simulink model "vipcodec"  (Simulink 7.7)
settings: Solver=FixedStepDiscrete  StartTime=0.0  StopTime=inf  RelTol=1e-3
undefined symbols (not defined in the file or in its folder): get, gray, M, N, rsgenpoly, sz
libraries: vipmisc x12, commutil2 x6, dspsigops x4, dspmtrx3 x4, vipsnks x3, commcnvintrlv2 x2, commblkcod2 x2, commcnvcod2 x2, viptransforms x2, viputilities x2, dspxfrm3 x2, commdigbbndam3 x2
settings Model: Creator=navan  LastModifiedBy=katsikas  CovMetricSettings=d  ExtModeAutoUpdateStatusClock=off
settings DataIOCC: SaveOutput=off  SaveTime=off  SignalLoggingName=logsOut
settings OptimizationCC: InlineParams=on  InlineInvariantSignals=on  InitFltsAndDblsToZero=on  EfficientMapNaN2IntZero=off  BufferReusableBoundary=off
settings DebuggingCC: SaveWithParameterizedLinksMsg=none  CheckExecutionContextPreStartOutputMsg=on  CheckExecutionContextRuntimeOutputMsg=on  SignalResolutionControl=TryResolveAllWithWarning  SolverPrmCheckMsg=none  MultiTaskDSMMsg=warning  MultiTaskCondExecSysMsg=none  BusObjectLabelMismatch=none  StrictBusMsg=None
settings HardwareCC: TargetBitPerLong=64  TargetBitPerPointer=64  TargetEndianess=LittleEndian  TargetWordSize=64  TargetHWDeviceType=Generic->MATLAB Host Computer  ProdEqTarget=off
settings ModelReferenceCC: UpdateModelReferenceTargets=IfOutOfDate
settings SFSimCC: SimParseCustomCode=off
settings RTWCC: IncludeERTFirstTime=on
settings GRTTargetCC: TargetFcnLib=ansi_tfl_tmw.mat

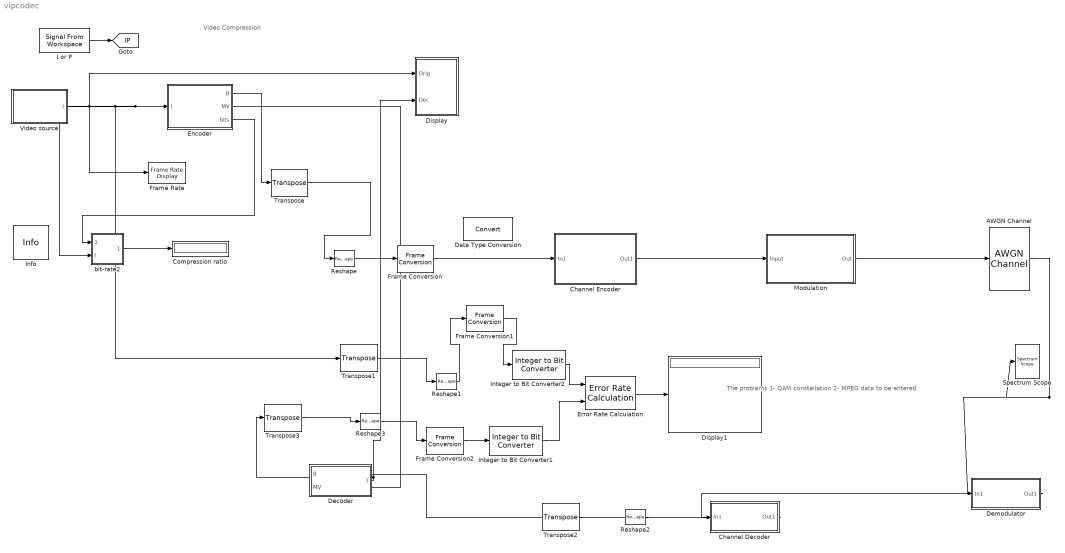
== system vipcodec ==
  note: Video Compression
  note: The problems
      | 1- QAM constellation
      | 2- MPEG data to be entered
  AWGN Channel : commchan3/AWGN Channel  SystemSampleTime=-1  InputProcessing=Inherited (this choice will be removed - see release notes)  seed=67  noiseMode="Signal to noise ratio  (SNR)"  EbNodB=10  EsNodB=10  SNRdB=10  bitsPerSym=1  Ps=1/2048  Tsym=1  variance=1
  Channel Decoder : Subsystem
  Channel Encoder : Subsystem
  Compression ratio : Display
  Data Type Conversion : DataTypeConversion
  Decoder : Subsystem
  Demodulator : Subsystem
  Display : Subsystem
  Display1 : Display
  Encoder : Subsystem
  Error Rate Calculation : commsink2/Error Rate Calculation  N=0  st_delay=0  cp_mode=Entire frame  subframe=[]  PMode=Port  WsName=ErrorVec  RsMode2=off  stop=off  numErr=100  maxBits=1e6
  Frame Conversion : FrameConversion
  Frame Conversion1 : FrameConversion
  Frame Conversion2 : FrameConversion
  Frame Rate : vipsnks/Frame Rate Display  UpdateRate=10
  I or P : dspsrcs4/Signal From Workspace  SystemSampleTime=-1  X=logical([0 0 1])  Ts=1/30  nsamps=1  OutputAfterFinalValue=Cyclic repetition  ignoreOrWarnInputAndFrameLengths=off
  Info : vipmisc/Info  SystemSampleTime=-1
  Integer to Bit Converter1 : commutil2/Integer to Bit Converter  nbits=8  signedInputValues=Unsigned  bitOrder=MSB first  outDtype=double
  Integer to Bit Converter2 : commutil2/Integer to Bit Converter  nbits=8  signedInputValues=Unsigned  bitOrder=MSB first  outDtype=double
  Modulation : Subsystem
  Reshape : Reshape  OutputDimensionality=Column vector (2-D)
  Reshape1 : Reshape  OutputDimensionality=Column vector (2-D)
  Reshape2 : Reshape  OutputDimensionality=Customize  OutputDimensions=[10,105]
  Reshape3 : Reshape  OutputDimensionality=Column vector (2-D)
  Spectrum Scope : dspsnks4/Spectrum Scope  SystemSampleTime=-1  ScopeProperties=on  Domain=Frequency  HorizSpan=1  UseBuffer=off  BufferSize=128  Overlap=64  TreatMby1Signals=One channel  inpFftLenInherit=off  FFTlength=128  numAvg=2  DisplayProperties=off  AxisGrid=on  Memory=off  FrameNumber=on  AxisLegend=off  AxisZoom=off  OpenScopeAtSimStart=on  OpenScopeImmediately=off  FigPos=get(0,'defaultfigureposition')  AxisProperties=off  XUnits=Hertz  XRange=[0...Fs/2]  XDisplay=0  InheritXIncr=on  XIncr=1.0  XLabel=Samples  XLimit=Auto  YUnits=dB  XMax=1  XMin=0  YLabel=Magnitude-squared, dB  LineProperties=off  wintypeSpecScope=Hann  RsSpecScope=50  betaSpecScope=5  winsampSpecScope=Periodic  XAxisParamsVer=6.8  isFrameUpgraded=on
      settings: YMin=-10  YMax=10
  Transpose{,1..3} (4 alike) : dspmtrx3/Transpose  SystemSampleTime=-1  Hermitian=off  overflowFlag=off
  Video source : Subsystem
  bit-rate2 : Subsystem
  tag scope: IP=global
  wires:
  Encoder/2(MV) -> Decoder/2(MV)
  Video source/1(I) -> Display/1(Orig), Encoder/1(I), bit-rate2/2(I), Transpose1/1, Frame Rate/1
  I or P/1 -> [IP]
  Encoder/3(bits) -> bit-rate2/1(bits)
  bit-rate2/1(ratio) -> Compression ratio/1
  AWGN Channel/1 -> Spectrum Scope/1, Demodulator/1(In1)
  Error Rate Calculation/1 -> Display1/1
  Modulation/1(Out) -> AWGN Channel/1
  Channel Encoder/1(Out1) -> Modulation/1(Input)
  Demodulator/1(Out1) -> Channel Decoder/1(In1)
  Integer to Bit Converter1/1 -> Error Rate Calculation/2
  Encoder/1(B) -> Transpose/1
  Transpose/1 -> Reshape/1
  Reshape/1 -> Frame Conversion/1
  Transpose1/1 -> Reshape1/1
  Decoder/1(I) -> Display/2(Dec), Transpose3/1
  Integer to Bit Converter2/1 -> Error Rate Calculation/1
  Reshape1/1 -> Frame Conversion1/1
  Frame Conversion1/1 -> Integer to Bit Converter2/1
  Channel Decoder/1(Out1) -> Reshape2/1
  Reshape2/1 -> Transpose2/1
  Transpose2/1 -> Decoder/1(B)
  Transpose3/1 -> Reshape3/1
  Reshape3/1 -> Frame Conversion2/1
  Frame Conversion2/1 -> Integer to Bit Converter1/1
  Frame Conversion/1 -> Channel Encoder/1(In1)

== system vipcodec/Channel Decoder ==
  In1 : Inport
  Bit to Integer Converter1 : commutil2/Bit to Integer Converter  nbits=8  bitOrder=MSB first  signedOutputValues=Unsigned  outDtype=uint32  outDtypeSigned=Inherit via internal rule
  Convolutional Deinterleaver : commcnvintrlv2/Convolutional Deinterleaver  SystemSampleTime=-1  N=15  B=15  ic=0
  Integer-Output RS Decoder : commblkcod2/Integer-Output RS Decoder  n=225  k=105  specPrimPoly=off  prPoly=[1 0 1 1]  specGenPoly=off  genPoly=rsgenpoly(7,3)  specPuncture=off  punctVec=[ones(2,1); zeros(2,1)]  specErasurePort=off  showNumErr=off
  Viterbi Decoder : commcnvcod2/Viterbi Decoder  trellis=poly2trellis(7, [171 133])  isPunctured=off  punctureVector=[1; 1; 0; 1; 0; 1]  erasures=off  dectype=Unquantized  runSigValErrCheck=off  nsdecb=4  smWordLength=16  tbdepth=34  opmode=Continuous  reset=off  outDataType=boolean
  Out1 : Outport
  wires:
  Viterbi Decoder/1 -> Bit to Integer Converter1/1
  Bit to Integer Converter1/1 -> Convolutional Deinterleaver/1
  Convolutional Deinterleaver/1 -> Integer-Output RS Decoder/1
  In1/1 -> Viterbi Decoder/1
  Integer-Output RS Decoder/1 -> Out1/1

== system vipcodec/Channel Encoder ==
  In1 : Inport
  Convolutional Encoder : commcnvcod2/Convolutional Encoder  trellis=poly2trellis(7, [171 133])  opMode=Continuous  DelayedResetAction=off  hasIniStPort=off  hasFinStPort=off  usePuncVector=off  punctureVector=[1; 1; 0; 1; 0; 1]  reset=Unused parameter value
  Convolutional Interleaver : commcnvintrlv2/Convolutional Interleaver  SystemSampleTime=-1  N=45  B=50  ic=0
  Integer to Bit Converter : commutil2/Integer to Bit Converter  nbits=8  signedInputValues=Unsigned  bitOrder=MSB first  outDtype=double
  Integer-Input RS Encoder : commblkcod2/Integer-Input RS Encoder  n=225  k=105  specPrimPoly=off  prPoly=[1 0 1 1]  specGenPoly=off  genPoly=rsgenpoly(7,3)  specPuncture=off  punctVec=[ones(2,1); zeros(2,1)]
  Out1 : Outport
  wires:
  Integer-Input RS Encoder/1 -> Convolutional Interleaver/1
  Convolutional Interleaver/1 -> Integer to Bit Converter/1
  Integer to Bit Converter/1 -> Convolutional Encoder/1
  Convolutional Encoder/1 -> Out1/1
  In1/1 -> Integer-Input RS Encoder/1

== system vipcodec/Decoder ==
  B : Inport
  MV : Inport  Port=2
  Block Processing : Subsystem  DialogController=vipDDGCreate  DialogControllerArgs=DataTag1  TreatAsAtomicUnit=on  mask(Block processing){NumI=3, NumO=1, Blocksize={[15 1],[46 46],[1 2]}, Overlapsize={[0 0],[30 30],[0 0]}, Traverse=Row-wise}
      mask prompts: NumI "Number of inputs:"; NumO "Number of outputs:"; Blocksize "Block size:"; Overlapsize "Overlap size:"; Traverse "Order of traversing:"
      mask help:
      | Repeat a user-specified operation on submatrices of the input matrix.
      |
      | This block extracts submatrices of a user-specified size from the input matrix. It sends each submatrix to a subsystem for processing, and then reassembles each subsystem output into the output matrix.
      |
      | Use the Block size and Overlap size parameters to specify the size and overlap of each submatrix in cell array format.
      settings: CopyFcn=set_param(gcb,'LinkStatus','none');
      mask Help: web(vipbhelp('Block Processing'));
      mask StyleString: edit,edit,edit,edit,popup(Row-wise|Column-wise)
      mask Display: disp('Block\n processing');
  Delay and pad : Subsystem
  I : Outport
  wires:
  B/1 -> Block Processing/1(In)
  Delay and pad/1(Out1) -> Block Processing/2(In2)
  MV/1 -> Block Processing/3(In3)
  Block Processing/1(Out) -> Delay and pad/1(In1), I/1
  [IP] -> Block Processing/4(ip)

== system vipcodec/Demodulator ==
  In1 : Inport
  Integer to Bit Converter3 : commutil2/Integer to Bit Converter  nbits=8  signedInputValues=Unsigned  bitOrder=MSB first  outDtype=double
  OFDM Receiver : Subsystem
      mask Display: disp('OFDM\nReceiver')
  Rectangular QAM Demodulator Baseband : commdigbbndam3/Rectangular QAM Demodulator Baseband  M=512  PowType=Min. distance between symbols  MinDist=2  AvgPow=1  PeakPow=1  Ph=0  Dec=Binary  Mapping=[0:15]  OutType=Integer  DecType=Hard decision  VarSource=Dialog  Variance=1  outDtype1=Inherit via internal rule  outDtype2=Inherit via internal rule  derotateFactorWordLen=16  denormFactorWordLen=16  prodOutWordLen=32  prodOutRoundingMode=Floor  prodOutOverflowMode=Wrap  sumWordLen=32
  Out1 : Outport
  wires:
  In1/1 -> OFDM Receiver/1(Received signal)
  OFDM Receiver/1(OFDM Spectrum) -> Rectangular QAM Demodulator Baseband/1
  Rectangular QAM Demodulator Baseband/1 -> Integer to Bit Converter3/1
  Integer to Bit Converter3/1 -> Out1/1

== system vipcodec/Display ==
  Orig : Inport
  Dec : Inport  Port=2
  Decoded : vipsnks/Video Viewer  inputType=Obsolete7b  imagePorts=One multidimensional signal  useColorMap=off  colormapValue=gray(256)  specRange=off  minInputVal=0  maxInputVal=255  FigPos=[769 486 160 128]  AxisZoom=on  trueSizedOnce=on  OpenAtMdlStart=on
  Original : vipsnks/Video Viewer  inputType=Obsolete7b  imagePorts=One multidimensional signal  useColorMap=off  colormapValue=gray(256)  specRange=off  minInputVal=0  maxInputVal=255  FigPos=[766 270 160 128]  AxisZoom=on  trueSizedOnce=on  OpenAtMdlStart=on
  wires:
  Orig/1 -> Original/1
  Dec/1 -> Decoded/1

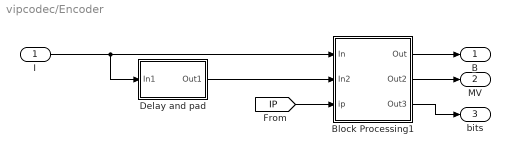
== system vipcodec/Encoder ==
  I : Inport
  Block Processing1 : Subsystem  DialogController=vipDDGCreate  DialogControllerArgs=DataTag5  TreatAsAtomicUnit=on  mask(Block processing){NumI=2, NumO=3, Blocksize={[16 16],[46 46]}, Overlapsize={[0 0],[30 30]}, Traverse=Row-wise}
      mask prompts: NumI "Number of inputs:"; NumO "Number of outputs:"; Blocksize "Block size:"; Overlapsize "Overlap size:"; Traverse "Order of traversing:"
      mask help:
      | Repeat a user-specified operation on submatrices of the input matrix.
      |
      | This block extracts submatrices of a user-specified size from the input matrix. It sends each submatrix to a subsystem for processing, and then reassembles each subsystem output into the output matrix.
      |
      | Use the Block size and Overlap size parameters to specify the size and overlap of each submatrix in cell array format.
      settings: CopyFcn=set_param(gcb,'LinkStatus','none');
      mask Help: web(vipbhelp('Block Processing'));
      mask StyleString: edit,edit,edit,edit,popup(Row-wise|Column-wise)
      mask Display: disp('Block\n processing');
  Delay and pad : Subsystem
  B : Outport
  MV : Outport  Port=2
  bits : Outport  Port=3
  wires:
  I/1 -> Delay and pad/1(In1), Block Processing1/1(In)
  Block Processing1/1(Out) -> B/1
  Delay and pad/1(Out1) -> Block Processing1/2(In2)
  Block Processing1/2(Out2) -> MV/1
  Block Processing1/3(Out3) -> bits/1
  [IP] -> Block Processing1/3(ip)

== system vipcodec/Modulation ==
  Input : Inport
  Bit to Integer Converter : commutil2/Bit to Integer Converter  nbits=8  bitOrder=MSB first  signedOutputValues=Unsigned  outDtype=Inherit via internal rule  outDtypeSigned=Inherit via internal rule
  OFDM Transmitter : Subsystem
      mask Display: disp('OFDM\nTransmitter')
  Rectangular QAM Modulator Baseband : commdigbbndam3/Rectangular QAM Modulator Baseband  M=256  InType=Integer  Enc=Binary  Mapping=[0:15]  PowType=Min. distance between symbols  MinDist=2  AvgPow=1  PeakPow=1  Ph=0  outDtype=double  outWordLen=16  outUDDataType=sfix(16)  outFracLenMode=Best precision  outFracLen=15
  Out : Outport
  wires:
  Bit to Integer Converter/1 -> Rectangular QAM Modulator Baseband/1
  Rectangular QAM Modulator Baseband/1 -> OFDM Transmitter/1(In)
  Input/1 -> Bit to Integer Converter/1
  OFDM Transmitter/1(Out) -> Out/1

== system vipcodec/Video source ==
  Image Data Type Conversion1 : vipconversions/Image Data Type Conversion  outDT=single  isSigned=on  wordLen=16  numFracBits=0
  Read Binary File : vipsrcs/Read Binary File  FileName=vipmen.bin  loopOrNot=on  numLoops=inf  VideoFormat=Custom  FOURCC=I420  BitStreamFormat=Planar  NumOutputs=3  ComponentOrder=[1 2 3]  Interlaced=off  LineOrdering=Top line first  Ts=1/30  Component1=Y'  Component2=Cb  Component3=Cr  Component4=Alpha  Bits1=8  Bits2=8  Bits3=8  Bits4=8  Rows1=120  Rows2=60  Rows3=60  Rows4=288  Cols1=160  Cols2=80  Cols3=80  Cols4=352  YRows=288  YCols=352  SignedOutput=off  FileEndian=Little endian  OutputEOF=off
  Selector2 : Selector  NumberOfDimensions=2  IndexMode=Zero-based  InputPortWidth=3  IndexOptions=Starting index (dialog),Starting index (dialog)  Indices=0,0  OutputSizes=112,160
  Terminator : Terminator
  Terminator1 : Terminator
  I : Outport
  wires:
  Image Data Type Conversion1/1 -> Selector2/1
  Selector2/1 -> I/1
  Read Binary File/1 -> Image Data Type Conversion1/1
  Read Binary File/2 -> Terminator/1
  Read Binary File/3 -> Terminator1/1

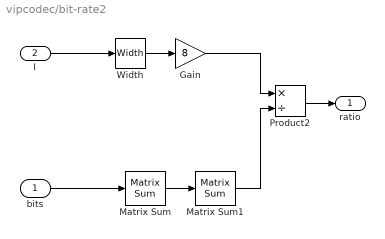
== system vipcodec/bit-rate2 ==
  bits : Inport
  I : Inport  Port=2
  Gain : Gain  Gain=8
  Matrix Sum : dspobslib/Matrix Sum  Dim=Columns  roundingMode=Floor  overflowMode=off
  Matrix Sum1 : dspobslib/Matrix Sum  Dim=Rows  roundingMode=Floor  overflowMode=off
  Product2 : Product  Inputs=*/  RndMeth=Zero
  Width : Width
  ratio : Outport
  wires:
  Product2/1 -> ratio/1
  I/1 -> Width/1
  Matrix Sum/1 -> Matrix Sum1/1
  bits/1 -> Matrix Sum/1
  Matrix Sum1/1 -> Product2/2
  Width/1 -> Gain/1
  Gain/1 -> Product2/1

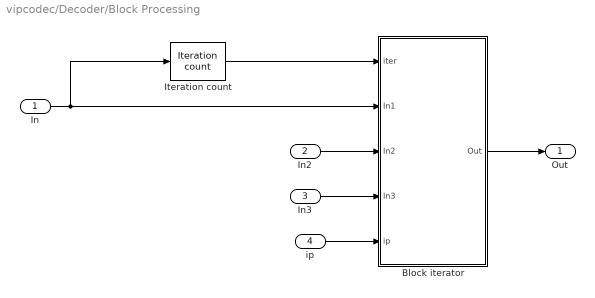
== system vipcodec/Decoder/Block Processing ==
  In : Inport
  In2 : Inport  Port=2
  In3 : Inport  Port=3
  ip : Inport  Port=4
  Block iterator : Subsystem
      settings: CopyFcn=set_param(gcb,'ReferenceBlock','');
  Iteration count : vipmisc/Iteration count  NumI=1  blksize=Blocksize{1}  ovlpsize=Overlapsize{1}
  Out : Outport
  wires:
  Iteration count/1 -> Block iterator/1(iter)
  In/1 -> Iteration count/1, Block iterator/2(In1)
  Block iterator/1(Out) -> Out/1
  In2/1 -> Block iterator/3(In2)
  In3/1 -> Block iterator/4(In3)
  ip/1 -> Block iterator/5(ip)

== system vipcodec/Decoder/Delay and pad ==
  In1 : Inport
  2-D Pad : viputilities/Image Pad  method=Constant  valSrc=Specify via dialog  value=0  spec=Pad size  rowDirection=Both left and right  outRowsMode=User-specified  rowSize=15  outColSize=10  colDirection=Both top and bottom  outColsMode=User-specified  colSize=15  outRowSize=12  trunc_flag=None
  Delay : dspsigops/Delay  InputProcessing=Inherited (this choice will be removed - see release notes)  dly_unit=Samples  delay=1  ic_detail=off  dif_ic_for_ch=off  dif_ic_for_dly=off  ic=0  reset_popup=None
  Out1 : Outport
  wires:
  Delay/1 -> 2-D Pad/1
  In1/1 -> Delay/1
  2-D Pad/1 -> Out1/1

== system vipcodec/Demodulator/OFDM Receiver ==
  Received signal : Inport
  FFT : dspxfrm3/FFT  CompMethod=Table lookup  TableOpt=NEW  TableOptActive=Speed  BitRevOrder=off  InheritFFTLength=on  FFTLength=64  RowConvenienceOn=on  SkipNorm=off  firstCoeffMode=Specify word length  firstCoeffWordLength=16  firstCoeffFracLength=15  firstCoeffDataTypeStr=fixdt(1,16)  firstCoeffLastDataTypeStr=fixdt(1,16)  outputMin=[]  outputMax=[]  accumDataTypeStr=Inherit: Same as product output  accumLastDataTypeStr=Inherit: Same as product output  roundingMode=Floor  overflowMode=off
  Frame Conversion : FrameConversion
  Remove zero pad from OFDM : Subsystem
      mask Display: disp('Remove zero\npad from OFDM');
  OFDM Spectrum : Outport
  wires:
  Remove zero pad from OFDM/1(Out1) -> OFDM Spectrum/1
  Received signal/1 -> FFT/1
  FFT/1 -> Frame Conversion/1
  Frame Conversion/1 -> Remove zero pad from OFDM/1(In1)

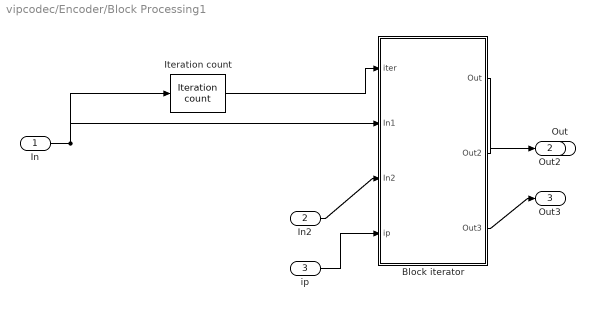
== system vipcodec/Encoder/Block Processing1 ==
  In : Inport
  In2 : Inport  Port=2
  ip : Inport  Port=3
  Block iterator : Subsystem
      settings: CopyFcn=set_param(gcb,'ReferenceBlock','');
  Iteration count : vipmisc/Iteration count  NumI=1  blksize=Blocksize{1}  ovlpsize=Overlapsize{1}
  Out : Outport
  Out2 : Outport  Port=2
  Out3 : Outport  Port=3
  wires:
  Iteration count/1 -> Block iterator/1(iter)
  In/1 -> Iteration count/1, Block iterator/2(In1)
  Block iterator/1(Out) -> Out/1
  In2/1 -> Block iterator/3(In2)
  Block iterator/2(Out2) -> Out2/1
  Block iterator/3(Out3) -> Out3/1
  ip/1 -> Block iterator/4(ip)

== system vipcodec/Encoder/Delay and pad ==
  In1 : Inport
  2-D Pad : viputilities/Image Pad  method=Constant  valSrc=Specify via dialog  value=0  spec=Pad size  rowDirection=Both left and right  outRowsMode=User-specified  rowSize=15  outColSize=10  colDirection=Both top and bottom  outColsMode=User-specified  colSize=15  outRowSize=12  trunc_flag=None
  Delay : dspsigops/Delay  InputProcessing=Inherited (this choice will be removed - see release notes)  dly_unit=Samples  delay=1  ic_detail=off  dif_ic_for_ch=off  dif_ic_for_dly=off  ic=0  reset_popup=None
  Out1 : Outport
  wires:
  In1/1 -> Delay/1
  Delay/1 -> 2-D Pad/1
  2-D Pad/1 -> Out1/1

== system vipcodec/Modulation/OFDM Transmitter ==
  In : Inport
  IFFT : dspxfrm3/IFFT  CompMethod=Table lookup  TableOpt=HYBRID  TableOptActive=Speed  BitRevOrder=off  cs_in=off  SkipNorm=on  InheritFFTLength=on  FFTLength=64  mode=Complex  outSamplingMode=Frame based  RowConvenienceOn=on  firstCoeffMode=User-defined  firstCoeffWordLength=16  firstCoeffFracLength=15  firstCoeffDataTypeStr=fixdt(1,16)  firstCoeffLastDataTypeStr=fixdt(1,16)  outputMin=[]  outputMax=[]  accumDataTypeStr=Inherit: Same as product output  accumLastDataTypeStr=Inherit: Same as product output  roundingMode=Floor  overflowMode=off
  Zero pad for OFDM : Subsystem
      mask Display: disp('Zero pad\nfor OFDM');
  Out : Outport
  wires:
  IFFT/1 -> Out/1
  In/1 -> Zero pad for OFDM/1(In1)
  Zero pad for OFDM/1(Out1) -> IFFT/1

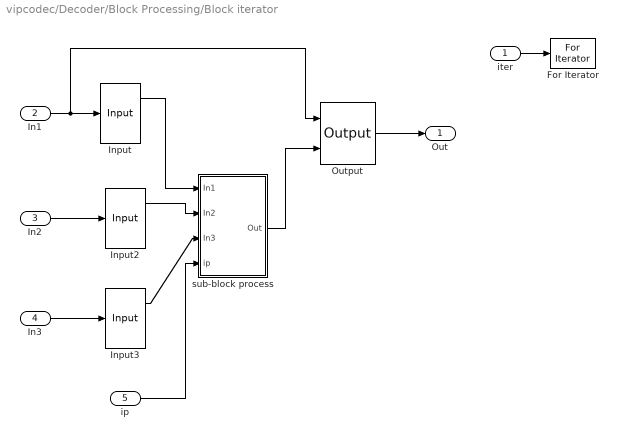
== system vipcodec/Decoder/Block Processing/Block iterator ==
  iter : Inport
  In1 : Inport  Port=2
  In2 : Inport  Port=3
  In3 : Inport  Port=4
  ip : Inport  Port=5
  For Iterator : ForIterator  IterationSource=external  IterationLimit=(sz(1)/M)*(sz(2)/N)  ShowIterationPort=off  IndexMode=Zero-based  IterationVariableDataType=double
  Input : vipmisc/Input  SystemSampleTime=-1  Blocksize=Blocksize{1}  Overlapsize=Overlapsize{1}  tverse=Row-wise
  Input2 : vipmisc/Input  SystemSampleTime=-1  Blocksize=Blocksize{2}  Overlapsize=Overlapsize{2}  tverse=Row-wise
  Input3 : vipmisc/Input  SystemSampleTime=-1  Blocksize=Blocksize{3}  Overlapsize=Overlapsize{3}  tverse=Row-wise
  Output : vipmisc/Output  SystemSampleTime=-1  Blocksize=Blocksize{1}  Overlapsize=Overlapsize{1}  tverse=Row-wise
  sub-block process : Subsystem
  Out : Outport
  wires:
  iter/1 -> For Iterator/1
  In1/1 -> Output/1, Input/1
  Output/1 -> Out/1
  sub-block process/1(Out) -> Output/2
  Input/1 -> sub-block process/1(In1)
  In2/1 -> Input2/1
  Input2/1 -> sub-block process/2(In2)
  In3/1 -> Input3/1
  Input3/1 -> sub-block process/3(In3)
  ip/1 -> sub-block process/4(ip)

== system vipcodec/Demodulator/OFDM Receiver/Remove zero pad from OFDM ==
  In1 : Inport
  Selector : Selector  NumberOfDimensions=2  InputPortWidth=2048  IndexOptions=Index vector (dialog),Select all  Indices=[1:2250 5943:8192],1  OutputSizes=1,1
  Out1 : Outport
  wires:
  In1/1 -> Selector/1
  Selector/1 -> Out1/1

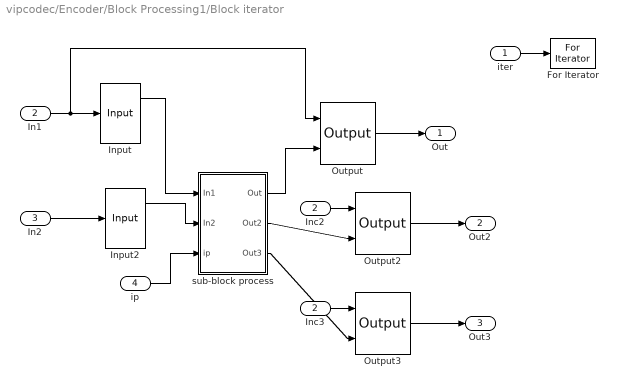
== system vipcodec/Encoder/Block Processing1/Block iterator ==
  iter : Inport
  In1 : Inport  Port=2
  In2 : Inport  Port=3
  ip : Inport  Port=4
  For Iterator : ForIterator  IterationSource=external  IterationLimit=(sz(1)/M)*(sz(2)/N)  ShowIterationPort=off  IndexMode=Zero-based  IterationVariableDataType=double
  Inc2 : InportShadow  Port=2
  Inc3 : InportShadow  Port=2
  Input : vipmisc/Input  SystemSampleTime=-1  Blocksize=Blocksize{1}  Overlapsize=Overlapsize{1}  tverse=Row-wise
  Input2 : vipmisc/Input  SystemSampleTime=-1  Blocksize=Blocksize{2}  Overlapsize=Overlapsize{2}  tverse=Row-wise
  Output : vipmisc/Output  SystemSampleTime=-1  Blocksize=Blocksize{1}  Overlapsize=Overlapsize{1}  tverse=Row-wise
  Output2 : vipmisc/Output  SystemSampleTime=-1  Blocksize=Blocksize{1}  Overlapsize=Overlapsize{1}  tverse=Row-wise
  Output3 : vipmisc/Output  SystemSampleTime=-1  Blocksize=Blocksize{1}  Overlapsize=Overlapsize{1}  tverse=Row-wise
  sub-block process : Subsystem
  Out : Outport
  Out2 : Outport  Port=2
  Out3 : Outport  Port=3
  wires:
  iter/1 -> For Iterator/1
  In1/1 -> Output/1, Input/1
  Output/1 -> Out/1
  sub-block process/1(Out) -> Output/2
  Input/1 -> sub-block process/1(In1)
  In2/1 -> Input2/1
  Input2/1 -> sub-block process/2(In2)
  Inc2/1 -> Output2/1
  Output2/1 -> Out2/1
  sub-block process/2(Out2) -> Output2/2
  Inc3/1 -> Output3/1
  Output3/1 -> Out3/1
  sub-block process/3(Out3) -> Output3/2
  ip/1 -> sub-block process/3(ip)

== system vipcodec/Modulation/OFDM Transmitter/Zero pad for OFDM ==
  In1 : Inport
  Selector : Selector  NumberOfDimensions=2  InputPortWidth=2048  IndexOptions=Index vector (dialog),Select all  Indices="[1:2250 4501:8192  2251:4500],1"  OutputSizes=1,1
  Zero Pad : dspsigops/Pad  padAlong=Columns  dimsToPad=1  valSrc=Specify via dialog  padVal=0  spec=Output size  padNumOutRowsSpecMethod=User-specified  numOutRows=8192  padNumOutColsSpecMethod=User-specified  numOutCols=1  isVarDimsMode=off  padBeginning=0  padEnd=0  outSizeMode=User-specified  outSize=1  padSigAt=End  trunc_flag=None  roundingMode=Floor  overflowMode=off  truncOrWrapMode=Truncate  wrap_flag=None
  Out1 : Outport
  wires:
  In1/1 -> Zero Pad/1
  Selector/1 -> Out1/1
  Zero Pad/1 -> Selector/1

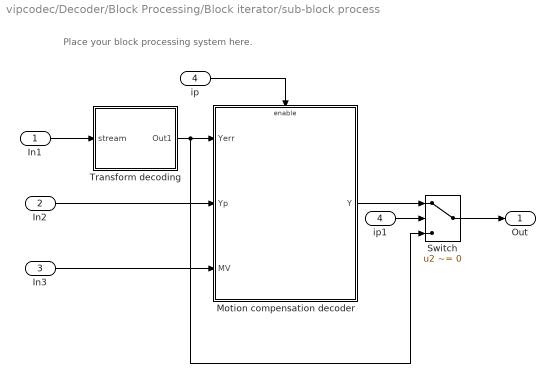
== system vipcodec/Decoder/Block Processing/Block iterator/sub-block process ==
  note: Place your block
      | processing system here.
  In1 : Inport
  In2 : Inport  Port=2
  In3 : Inport  Port=3
  ip : Inport  Port=4
  Motion compensation decoder : Subsystem
  Switch : Switch  Criteria=u2 ~= 0
  Transform decoding : Subsystem
  ip1 : InportShadow  Port=4
  Out : Outport
  wires:
  In1/1 -> Transform decoding/1(stream)
  Transform decoding/1(Out1) -> Motion compensation decoder/1(Yerr), Switch/3
  Motion compensation decoder/1(Y) -> Switch/1
  Switch/1 -> Out/1
  ip1/1 -> Switch/2
  In2/1 -> Motion compensation decoder/2(Yp)
  In3/1 -> Motion compensation decoder/3(MV)
  ip/1 -> Motion compensation decoder/Enable

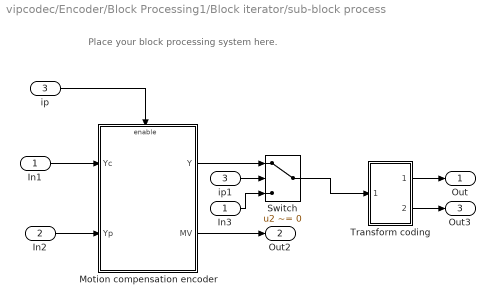
== system vipcodec/Encoder/Block Processing1/Block iterator/sub-block process ==
  note: Place your block
      | processing system here.
  In1 : Inport
  In2 : Inport  Port=2
  ip : Inport  Port=3
  In3 : InportShadow  Port=1
  Motion compensation encoder : Subsystem
  Switch : Switch  Criteria=u2 ~= 0
  Transform coding : Subsystem
  ip1 : InportShadow  Port=3
  Out : Outport
  Out2 : Outport  Port=2
  Out3 : Outport  Port=3
  wires:
  In1/1 -> Motion compensation encoder/1(Yc)
  In2/1 -> Motion compensation encoder/2(Yp)
  ip/1 -> Motion compensation encoder/Enable
  ip1/1 -> Switch/2
  In3/1 -> Switch/3
  Motion compensation encoder/1(Y) -> Switch/1
  Motion compensation encoder/2(MV) -> Out2/1
  Transform coding/1(stream) -> Out/1
  Transform coding/2(bits) -> Out3/1
  Switch/1 -> Transform coding/1(In1)

== system vipcodec/Decoder/Block Processing/Block iterator/sub-block process/Motion compensation decoder ==
  Yerr : Inport
  Yp : Inport  Port=2
  MV : Inport  Port=3
  Enable : EnablePort
  SelectMatch3 : Subsystem
  Sum5 : Sum  Inputs=|++
  Y : Outport
  wires:
  MV/1 -> SelectMatch3/2(Indx)
  Yp/1 -> SelectMatch3/1(Image)
  Sum5/1 -> Y/1
  SelectMatch3/1(Out) -> Sum5/1
  Yerr/1 -> Sum5/2

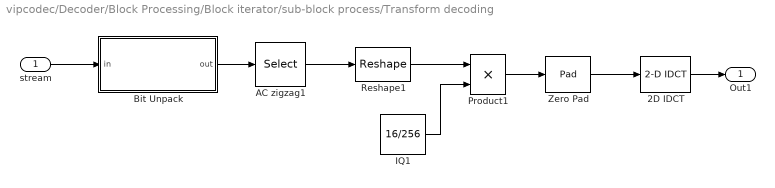
== system vipcodec/Decoder/Block Processing/Block iterator/sub-block process/Transform decoding ==
  stream : Inport
  2D IDCT : viptransforms/2-D IDCT  CompMethod=Table lookup  Dimension=0  TableOpt=Speed  BitRevOrder=off  SkipNorm=off  firstCoeffDataTypeStr=Inherit: Same word length as input  firstCoeffLastDataTypeStr=Inherit: Same word length as input  outputMin=[]  outputMax=[]  roundingMode=Floor  overflowMode=off
  AC zigzag1 : Selector  IndexOptions=Index vector (dialog)  Indices="[1     3     4    10    11    21    22    36     2     5     9    12    20    23    35    37     6     8    13    19    24    34    38    49     7    14    18    25    33    39    48    50    15    17    26    32    40    47    51     58    16    27    31    41    46    52    57    59    28    30    42    45     53    56    60    63    29    43    44    54    55    61    62    64]"  OutputSizes=1
  Bit Unpack : Stateflow chart  TreatAsAtomicUnit=on
  IQ1 : Constant  Value=16/256  VectorParams1D=off  OutDataTypeStr=Inherit: Inherit via back propagation
  Product1 : Product  SaturateOnIntegerOverflow=on  RndMeth=Zero  OutDataTypeStr=Inherit: Same as first input
  Reshape1 : Reshape  OutputDimensionality=Customize  OutputDimensions=[8,8]
  Zero Pad : dspsigops/Pad  padAlong=Columns and rows  dimsToPad=1  valSrc=Specify via dialog  padVal=0  spec=Output size  padNumOutRowsSpecMethod=User-specified  numOutRows=16  padNumOutColsSpecMethod=User-specified  numOutCols=16  isVarDimsMode=off  padBeginning=0  padEnd=0  outSizeMode=User-specified  outSize=1  padSigAt=End  trunc_flag=None  roundingMode=Floor  overflowMode=off  truncOrWrapMode=Truncate  wrap_flag=None
  Out1 : Outport
  wires:
  AC zigzag1/1 -> Reshape1/1
  Bit Unpack/1(out) -> AC zigzag1/1
  2D IDCT/1 -> Out1/1
  stream/1 -> Bit Unpack/1(in)
  Zero Pad/1 -> 2D IDCT/1
  Reshape1/1 -> Product1/1
  Product1/1 -> Zero Pad/1
  IQ1/1 -> Product1/2

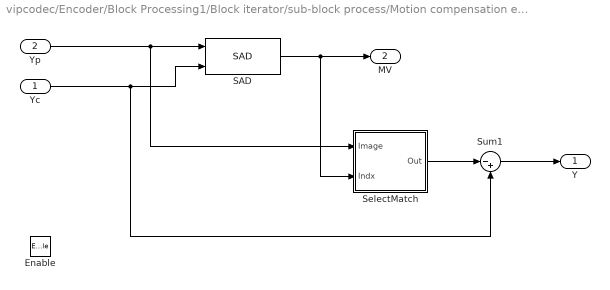
== system vipcodec/Encoder/Block Processing1/Block iterator/sub-block process/Motion compensation encoder ==
  Yc : Inport
  Yp : Inport  Port=2
  Enable : EnablePort
  SAD : vipobslib/SAD  output=Minimum SAD value index  method=Three-step  roi=off  invalidROI=Ignore  nearbyPel=off  nearbySize=3  roundingMode=Floor  overflowMode=off
  SelectMatch : Subsystem
  Sum1 : Sum  Inputs=|-+  OutDataTypeStr=Inherit: Same as first input
  Y : Outport
  MV : Outport  Port=2
  wires:
  SAD/1 -> SelectMatch/2(Indx), MV/1
  Sum1/1 -> Y/1
  SelectMatch/1(Out) -> Sum1/1
  Yc/1 -> SAD/2, Sum1/2
  Yp/1 -> SelectMatch/1(Image), SAD/1

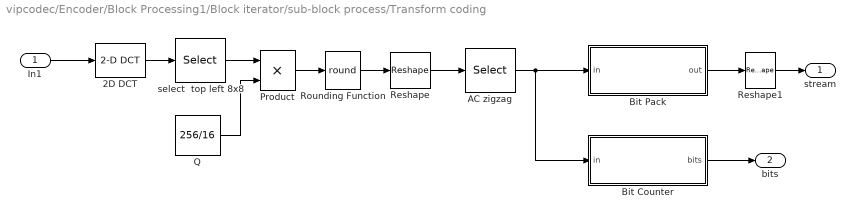
== system vipcodec/Encoder/Block Processing1/Block iterator/sub-block process/Transform coding ==
  In1 : Inport
  2D DCT : viptransforms/2-D DCT  CompMethod=Table lookup  Dimension=0  TableOpt=Speed  BitRevOrder=off  SkipNorm=off  firstCoeffDataTypeStr=Inherit: Same word length as input  firstCoeffLastDataTypeStr=Inherit: Same word length as input  outputMin=[]  outputMax=[]  roundingMode=Floor  overflowMode=off
  AC zigzag : Selector  IndexOptions=Index vector (dialog)  Indices="[0  8     1     2     9    16    24    17    10     3     4    11    18    25  32    40    33    26    19    12     5     6    13    20    27    34    41  48    56    49    42    35    28    21    14     7    15    22    29    36  43    50    57    58    51    44    37    30    23    31    38    45    52  59    60    53    46    39    47    54    61    62    55    63]+1"  OutputSizes=1
  Bit Counter : Stateflow chart  TreatAsAtomicUnit=on
  Bit Pack : Stateflow chart  TreatAsAtomicUnit=on
  Product : Product  SaturateOnIntegerOverflow=on  RndMeth=Zero  OutDataTypeStr=Inherit: Same as first input
  Q : Constant  Value=256/16  VectorParams1D=off  OutDataTypeStr=Inherit: Inherit via back propagation
  Reshape : Reshape  OutputDimensionality=Column vector (2-D)  OutputDimensions=[8,8]
  Reshape1 : Reshape  OutputDimensionality=Column vector (2-D)  OutputDimensions=[8,8]
  Rounding Function : Rounding  Operator=round
  select  top left 8x8 : Selector  NumberOfDimensions=2  IndexMode=Zero-based  IndexOptions=Starting index (dialog),Starting index (dialog)  Indices=0,0  OutputSizes=8,8
  stream : Outport
  bits : Outport  Port=2
  wires:
  Reshape/1 -> AC zigzag/1
  Reshape1/1 -> stream/1
  2D DCT/1 -> select  top left 8x8/1
  In1/1 -> 2D DCT/1
  AC zigzag/1 -> Bit Counter/1(in), Bit Pack/1(in)
  Product/1 -> Rounding Function/1
  Rounding Function/1 -> Reshape/1
  select  top left 8x8/1 -> Product/1
  Bit Counter/1(bits) -> bits/1
  Q/1 -> Product/2
  Bit Pack/1(out) -> Reshape1/1

== system vipcodec/Decoder/Block Processing/Block iterator/sub-block process/Motion compensation decoder/SelectMatch3 ==
  Image : Inport
  Indx : Inport  Port=2
  Selector3 : Selector  NumberOfDimensions=2  IndexMode=Zero-based  InputPortWidth=3  IndexOptions=Starting index (port),Starting index (port)  Indices=1,1  OutputSizes=16,16
  Selector4 : Selector  InputPortWidth=2  IndexOptions=Index vector (dialog)  Indices=1  OutputSizes=1
  Selector5 : Selector  InputPortWidth=2  IndexOptions=Index vector (dialog)  Indices=2  OutputSizes=1
  Out : Outport
  wires:
  Selector4/1 -> Selector3/2
  Selector5/1 -> Selector3/3
  Image/1 -> Selector3/1
  Indx/1 -> Selector4/1, Selector5/1
  Selector3/1 -> Out/1

== system vipcodec/Encoder/Block Processing1/Block iterator/sub-block process/Motion compensation encoder/SelectMatch ==
  Image : Inport
  Indx : Inport  Port=2
  Selector3 : Selector  NumberOfDimensions=2  IndexMode=Zero-based  InputPortWidth=3  IndexOptions=Starting index (port),Starting index (port)  Indices=1,1  OutputSizes=16,16
  Selector4 : Selector  InputPortWidth=2  IndexOptions=Index vector (dialog)  Indices=1  OutputSizes=1
  Selector5 : Selector  InputPortWidth=2  IndexOptions=Index vector (dialog)  Indices=2  OutputSizes=1
  Out : Outport
  wires:
  Selector3/1 -> Out/1
  Indx/1 -> Selector5/1, Selector4/1
  Image/1 -> Selector3/1
  Selector5/1 -> Selector3/3
  Selector4/1 -> Selector3/2

== matlab function Encoder/Block Processing1/Block iterator/sub-block process/Transform coding/Bit Pack ==
  data: in input double; out output uint32 size=15
function out=bitpack(in) 

% Pack output bits into given length using run length coding. The first 
% coefficient (DC) is coded using 32 bits. The AC coefficients are run 
% length coded using 4 bits for run and 8 bits for value. The output is uint32.

persistent prev_out;
if isempty(prev_out)
    prev_out = uint32(zeros(15,1));
end
    out=uint32(prev_out);
    % Bit Pack Routine  
    bitpos=int32(0); 
    Temp= uint32(0); 
    run =  uint32(0); 
    outpos = 2; 
    pval=single(0); 
    cval=single(0);
  
    numcoefs = 64;
    
    out1 =  int32(fix(in(1)));
    
    if out1>=-1   
       out(1) = uint32(out1);
    else
       out(1) = uint32(intmax('uint32') - uint32(abs(out1)) +uint32(2));
    end

    % ac coefficients
    % 4 bit - run length followed by 8 bit coef value  
    pval(:) = fix(in(2)+0.5);
    if (pval > 127),  pval(:) = 127; end % saturate  
    if (pval < -128), pval(:) = -128; end

    run(:) = 0;
    for i=(3): numcoefs   
        cval(:) = floor(in(i)+0.5); 
        if (pval == cval && run < 14)  
            run(:)=run(:)+1;
        else  
            [flag, bitpos, out, Temp, outpos] = putbits(bitpos, out, Temp, outpos, run, 4);
            if (~flag) 
                prev_out=out;
                return; 
            end

            if (pval > 127),  pval(:) = 127;  end % saturate  
            if (pval < -128), pval(:) = -128; end
            pval(:) = pval+128; % make positive  

            [flag, bitpos, out, Temp, outpos] = putbits(bitpos, out, Temp, outpos, uint32(pval), 8);
            if (~flag) 
                prev_out=out;
                return; 
            end

            run(:) = 0;
        end
        pval(:) = cval;
    end

    % last coefficient  
    [flag, bitpos, out, Temp, outpos] = putbits(bitpos, out, Temp, outpos, run, 4);
    if (~flag) 
        prev_out=out;
        return; 
    end

    if (pval > 127),  pval(:) = 127;  end % saturate 
    if (pval < -128), pval(:) = -128; end
    pval(:) = pval+128; % make positive 

    [flag, bitpos, out, Temp, outpos] = putbits(bitpos, out, Temp, outpos, pval, 8);
    if (~flag) 
        prev_out=out;
        return; 
    end

    [bitpos, out, Temp, outpos] = flushbits(bitpos, out, Temp, outpos);%#ok
    prev_out=out;
end

%%========================================================================
function [flag, bitposO, outO, TempO, outposO] = putbits(bitpos, out, Temp, outpos, val, bits)
     
    valIn = uint32(val);
    bitsIn=int32(bits);
    bitposO = int32(bitpos);
    outO = uint32(out);
    TempO = uint32(Temp);
    outposO = outpos;
    
    if (bitposO + bitsIn > 32)  
        bitsleft = int32(32 - bitposO);
        bval=uint32(0);
        bval(:) = bitshift(valIn, -(bitsIn-bitsleft)); 
        TempO(:) = bitor(TempO,bval); 
        outO(outposO) = TempO;
        outposO = outposO+1;
        if (outposO > length(out))  
            flag = 0;
            return;
        end
        TempO = uint32(0);
        bitposO(:) = int32(0);
        bitsIn(:) = bitsIn-bitsleft; 
        valIn(:)=bitshift(valIn, 32-bitsIn);  
        valIn(:)=bitshift(valIn, -(32-bitsIn)); 
    end
    valIn(:)=bitshift(valIn, (32-(bitsIn+(bitposO))));  
    TempO = bitor(TempO, valIn); 
    bitposO(:) = bitposO + bitsIn;
    flag=1;
end

%%========================================================================
function [bitposO, outO, TempO, outposO, out] = flushbits(bitpos, out, Temp, outpos)
 
    [flag, bitposO, outO, TempO, outposO] = putbits(bitpos, out, Temp, outpos, 15, 4);
    if (~flag) 
        return; 
    end
    if (outposO > length(out)+1), return; end
    outO(outposO) = TempO;
end

== matlab function Encoder/Block Processing1/Block iterator/sub-block process/Transform coding/Bit Counter ==
  data: in input double; bits output double
function bits = bitcounter(in)
% This bitcounter assumes that the input signal will be 
% huffman encoded and counts bits based on this assumption. Note 
% however that the Bit Pack and Bit Unpack blocks only perform
% run length encoding.

numacbits = 0;
run = 0;

dclen = [2, 3, 3, 3, 3, 3, 4, 5, 6, 7, 8, 9];

if (in(1) < 0) 
    dcval = uint32(-in(1)); 
else
    dcval = uint32(in(1)); 
end

for i=0:11
    if (dcval == 0) 
        break; 
    end
    dcval = uint32(bitshift(dcval,-1));
end
numdcbits = dclen(i+1) + i;

aclen = [2,  2,  3,  4,  5,  7,  8, 10, 16, 16,...
    4,  5,  7,  9, 11, 16, 16, 16, 16, 16,...
    5,  8, 10, 12, 16, 16, 16, 16, 16, 16,...
    6,  9, 12, 16, 16, 16, 16, 16, 16, 16,...
    6, 10, 16, 16, 16, 16, 16, 16, 16, 16,...
    7, 11, 16, 16, 16, 16, 16, 16, 16, 16,...
    7, 12, 16, 16, 16, 16, 16, 16, 16, 16,...
    8, 12, 16, 16, 16, 16, 16, 16, 16, 16,...
    9, 15, 16, 16, 16, 16, 16, 16, 16, 16,...
    9, 16, 16, 16, 16, 16, 16, 16, 16, 16,...
    9, 16, 16, 16, 16, 16, 16, 16, 16, 16,...
    10, 16, 16, 16, 16, 16, 16, 16, 16, 16,...
    10, 16, 16, 16, 16, 16, 16, 16, 16, 16,...
    11, 16, 16, 16, 16, 16, 16, 16, 16, 16,...
    16, 16, 16, 16, 16, 16, 16, 16, 16, 16,...
    16, 16, 16, 16, 16, 16, 16, 16, 16, 16];



for i=1:63
    if (in(i+1) == 0)
        run = run+1;
        if (i < 63)
            continue;
        end
    end
    
    if (in(i+1) < 0) 
        acval = uint32(-in(i+1)); 
    else
        acval = uint32(in(i+1));
    end

    for j=0:31
        if (acval == 0) 
            break; 
        end

        acval = uint32(bitshift(acval,-1));
    end
    
    while (run > 15)
        run = run-15;
        numacbits = numacbits+11;
    end

    numacbits = numacbits + aclen(run*10 + j+1) + j;
    run = 0;
end

if (run > 0) 
    numacbits = numacbits+4; 
end
     
bits = single(numacbits+numdcbits);

== matlab function Decoder/Block Processing/Block iterator/sub-block process/Transform decoding/Bit Unpack ==
  data: in input double; out output single size=64
function out=bitunpack(in)

% Unpack the bits packed by the bit pack block. If there are not enough 
% values in the packed stream the rest of the output is filled with zeros.

persistent prev_out;
if isempty(prev_out)
    prev_out = single(zeros(64,1));
end
    out = prev_out;
    cbits= int32(0); 
    inpos=2; 
    Temp = uint32(0); 
    run = uint32(0);
    val = uint32(0);
   
    numcoefs = 64;
    if bitget(in(1),32)%negative
        out(1)=-int32(intmax('uint32')- uint32(in(1))) - int32(1);
    else
        out(1)=int32(in(1));
    end
    
    % ac coefficients
    % 4 bit - run length followed by 8 bit coef value  
    i=2;
    while (i<=numcoefs)   
         
        [flag, cbits, inpos, Temp, run] = getbits(cbits, inpos, Temp, in, run, 4);
        if (~flag) 
            break; 
        end
        if (run == 15), break;   end % end of stream  
        
        [flag, cbits, inpos, Temp, val] = getbits(cbits, inpos, Temp, in, val, 8);
        if (~flag) 
            break; 
        end 
        
        for j= i: min(run+i, numcoefs)    
            out(j) = single(single(val)-128.0);  
        end
        i = i + double(run)+1;
    end

    % when we havent got all coefs in the stream 
    for i=i:numcoefs    
        out(i) = 0;
    end
    prev_out(:)=out;
end

%%=================================================
function [flag, cbitsO, inposO, TempO, valO] = getbits(cbits, inpos, Temp, in, val, bits)

    lval = uint32(0); 
    temp = uint32(0);
    cbitsO = int32(cbits);
    inposO = inpos;
    TempO = uint32(Temp);
    valO = uint32(val);
    inwidth = length(in);
    if (cbitsO < bits)  
        if (inposO > inwidth) 
            flag=0;
            return; 
        end

        lval(:) =  bitshift(TempO, -(32-cbitsO));  
        bits(:) = bits - cbitsO;
        TempO = in(inposO); inposO = inposO +1;  
        lval = bitshift(lval, bits);  
        cbitsO(:) = int32(32);
    end

    temp(:) = bitshift(TempO, -(32-bits));  
    TempO(:) = bitshift(TempO, bits);  
    valO(:) = bitor(lval, temp); 
    cbitsO(:) = cbitsO - bits;

    flag = 1;
end
